simulink model "overflow"  (R2017a)
settings: Solver=VariableStepAuto  StartTime=0.0  StopTime=10.0  RelTol=1e-3
libraries: simulink x1
settings Model: Creator=kando  LastModifiedBy=kando

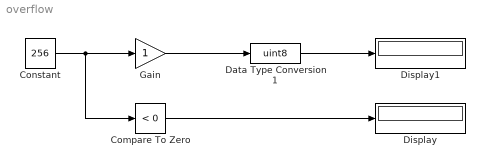
== system overflow ==
  Compare To Zero : simulink/Logic and Bit Operations/Compare To Zero  relop=<  OutDataTypeStr=uint8
  Constant : Constant  Value=256
  Data Type Conversion1 : DataTypeConversion  OutDataTypeStr=uint8
      settings: AttributesFormatString=|
      | saturateOverflow(%<SaturateOnIntegerOverflow>)
      | %<ConvertRealWorld>
  Display : Display
  Display1 : Display
  Gain : Gain  RndMeth=Round
      settings: AttributesFormatString=%<Gain>
  wires:
  Gain/1 -> Data Type Conversion1/1
  Constant/1 -> Compare To Zero/1, Gain/1
  Data Type Conversion1/1 -> Display1/1
  Compare To Zero/1 -> Display/1
